simulink model "main"  (R2015a)
settings: Solver=ode1  StartTime=0.0  StopTime=Inf  FixedStep=0.001  RelTol=1e-3
PostLoadFcn:
  | , if any(exist('dsrtsu_mdlpostloadfcn', 'file') == [2, 3, 6]), try dsrtsu_mdlpostloadfcn('Execute', bdroot); catch fprintf('Error in PostLoadFcn (dsrtsu_mdlpostloadfcn) for model "%s":\n %s\n', bdroot, lasterr); end, end,
libraries: rtilibm x3, simulink_extras x3
settings Model: DSRTSU_INTERNAL_RTI_VER=460  DSRTSU_INTERNAL_RTI_TYPE=rti1005  DSRTSU_INTERNAL_RTIFPGA=50  Creator=k19p1400a  LastModifiedBy=k19p1400a
settings OptimizationCC: BlockReduction=off  OptimizeBlockIOStorage=off  BufferReuse=off  GlobalBufferReuse=off  ExpressionFolding=off  LocalBlockOutputs=off
settings HardwareCC: ProdIntDivRoundTo=Zero  ProdEndianess=BigEndian  ProdHWDeviceType=Generic->Custom  TargetIntDivRoundTo=Zero  TargetEndianess=BigEndian  TargetHWDeviceType=Generic->Custom
settings RTWCC: SystemTargetFile=rti1005.tlc  MakeCommand=make_rti  TemplateMakefile=rti1005.tmf  Description=dSPACE DS1005 Hardware Platform
settings STFCustomTargetCC: GenerateSampleERTMain=off  ParMdlRefBuildCompliant=on  GeneratePreprocessorConditionals=Disable all  ERTCustomFileBanners=off  SupportNonInlinedSFcns=on  SupportVariableSizeSignals=off  MATLABClassNameForMDSCustomization=Simulink.SoftwareTarget.GRTCustomization  GRTInterface=on  SystemTargetFile=rti1005.tlc
settings GRTTargetCC: CompOptLevelCompliant=off  ConcurrentExecutionCompliant=off  CombineOutputUpdateFcns=off  MatFileLogging=off  CPPClassGenCompliant=off  GRTInterface=on  ExtModeMexFile=noextcomm

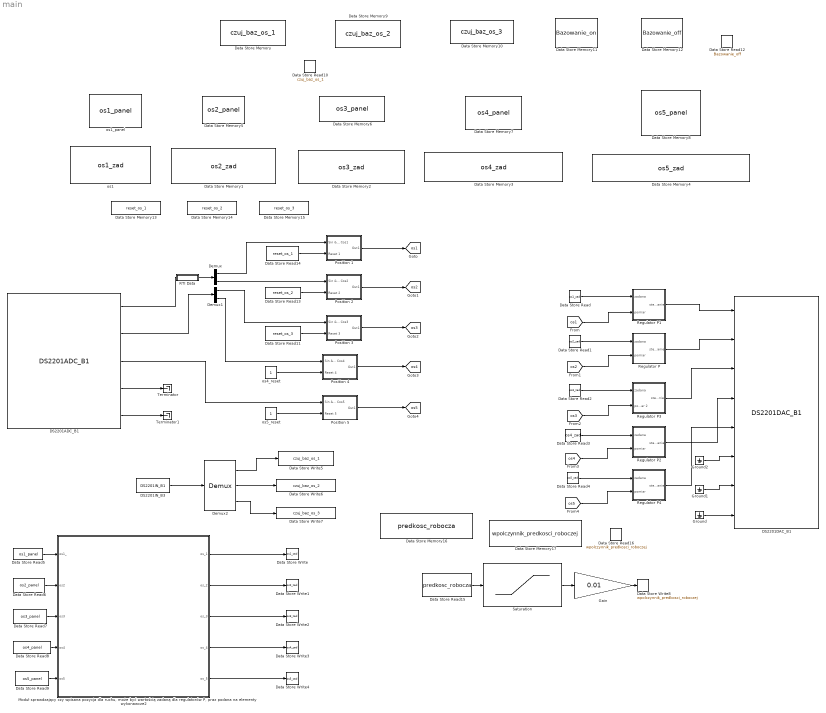
== system main ==
  DS2201ADC_B1 : rtilibm/DS2201/DS2201ADC_B1  BoardNo=1  channelNo1=[1 2 3 4]  channelNo2=[5 6 7 8]  channelNo3=[9 10]  channelNo4=-1  channelNo5=-1  DialogFcn=gui2201adc  UnitName={'DS2201ADC_B'}  UnitValues={ 1 }  DSProperties=struct('RTI',struct('Version',uint32(1),'BlockType',struct('isSLSource',uint8(1),'isSLSink',uint8(0),'isHWSource',uint8(1),'isHWSink',uint8(0),'isSetup',uint8(0),'isInline',uint8(1),'isNonInline',uint8(0),'isInterrupt',uint8(0),'isChannelwise',uint8(0)),'IOBoardType','DS2201','UnitType','ADC','Identifier','ADCMUX','DialogType','ML','BlockSet','NONE','SlaveProcessor','NONE'))
  DS2201DAC_B1 : rtilibm/DS2201/DS2201DAC_B1  BoardNo=1  IOErrorMode=[0 0]  InitValue=[0 0 0 0 0 0 0 0]  TermMode=[0 0 0 0 0 0 0 0]  TermValue=[0 0 0 0 0 0 0 0]  DialogFcn=gui2201dac  UnitName={'DS2201DAC_B'}  UnitValues={ 1 }  DSProperties=struct('RTI',struct('Version',uint32(1),'BlockType',struct('isSLSource',uint8(0),'isSLSink',uint8(1),'isHWSource',uint8(0),'isHWSink',uint8(1),'isSetup',uint8(0),'isInline',uint8(1),'isNonInline',uint8(0),'isInterrupt',uint8(0),'isChannelwise',uint8(0)),'IOBoardType','DS2201','UnitType','DAC','Identifier','DAC','DialogType','ML','BlockSet','NONE','SlaveProcessor','NONE'))
  DS2201IN_B3 : rtilibm/DS2201/DS2201IN_B1  BoardNo=3  ChannelNos=[1 2 3]  DialogFcn=gui2201in  UnitName={ 'DS2201IN_B' }  UnitValues={ 3 }  DSProperties=struct('RTI',struct('Version',uint32(1),'BlockType',struct('isSLSource',uint8(1),'isSLSink',uint8(0),'isHWSource',uint8(1),'isHWSink',uint8(0),'isSetup',uint8(0),'isInline',uint8(1),'isNonInline',uint8(0),'isInterrupt',uint8(0),'isChannelwise',uint8(0)),'IOBoardType','DS2201','UnitType','BIT','Identifier','BITIN','DialogType','ML','BlockSet','NONE','SlaveProcessor','NONE'))
  Data Store Memory : DataStoreMemory  DataStoreName=czuj_baz_os_1  ReadBeforeWriteMsg=warning  WriteAfterWriteMsg=warning  WriteAfterReadMsg=warning
  Data Store Memory1 : DataStoreMemory  DataStoreName=os2_zad  ReadBeforeWriteMsg=warning  WriteAfterWriteMsg=warning  WriteAfterReadMsg=warning
  Data Store Memory10 : DataStoreMemory  DataStoreName=czuj_baz_os_3  ReadBeforeWriteMsg=warning  WriteAfterWriteMsg=warning  WriteAfterReadMsg=warning
  Data Store Memory11 : DataStoreMemory  DataStoreName=Bazowanie_on  ReadBeforeWriteMsg=warning  WriteAfterWriteMsg=warning  WriteAfterReadMsg=warning  OutDataTypeStr=double
  Data Store Memory12 : DataStoreMemory  DataStoreName=Bazowanie_off  ReadBeforeWriteMsg=warning  WriteAfterWriteMsg=warning  WriteAfterReadMsg=warning  OutDataTypeStr=double
  Data Store Memory13 : DataStoreMemory  DataStoreName=reset_os_1  ReadBeforeWriteMsg=warning  WriteAfterWriteMsg=warning  WriteAfterReadMsg=warning
  Data Store Memory14 : DataStoreMemory  DataStoreName=reset_os_2  ReadBeforeWriteMsg=warning  WriteAfterWriteMsg=warning  WriteAfterReadMsg=warning
  Data Store Memory15 : DataStoreMemory  DataStoreName=reset_os_3  ReadBeforeWriteMsg=warning  WriteAfterWriteMsg=warning  WriteAfterReadMsg=warning
  Data Store Memory16 : DataStoreMemory  DataStoreName=predkosc_robocza  ReadBeforeWriteMsg=warning  WriteAfterWriteMsg=warning  WriteAfterReadMsg=warning
  Data Store Memory17 : DataStoreMemory  DataStoreName=wpolczynnik_predkosci_roboczej  ReadBeforeWriteMsg=warning  WriteAfterWriteMsg=warning  WriteAfterReadMsg=warning
  Data Store Memory2 : DataStoreMemory  DataStoreName=os3_zad  ReadBeforeWriteMsg=warning  WriteAfterWriteMsg=warning  WriteAfterReadMsg=warning
  Data Store Memory3 : DataStoreMemory  DataStoreName=os4_zad  ReadBeforeWriteMsg=warning  WriteAfterWriteMsg=warning  WriteAfterReadMsg=warning
  Data Store Memory4 : DataStoreMemory  DataStoreName=os5_zad  ReadBeforeWriteMsg=warning  WriteAfterWriteMsg=warning  WriteAfterReadMsg=warning
  Data Store Memory5 : DataStoreMemory  DataStoreName=os2_panel  ReadBeforeWriteMsg=warning  WriteAfterWriteMsg=warning  WriteAfterReadMsg=warning
  Data Store Memory6 : DataStoreMemory  DataStoreName=os3_panel  ReadBeforeWriteMsg=warning  WriteAfterWriteMsg=warning  WriteAfterReadMsg=warning
  Data Store Memory7 : DataStoreMemory  DataStoreName=os4_panel  ReadBeforeWriteMsg=warning  WriteAfterWriteMsg=warning  WriteAfterReadMsg=warning
  Data Store Memory8 : DataStoreMemory  DataStoreName=os5_panel  ReadBeforeWriteMsg=warning  WriteAfterWriteMsg=warning  WriteAfterReadMsg=warning
  Data Store Memory9 : DataStoreMemory  DataStoreName=czuj_baz_os_2  ReadBeforeWriteMsg=warning  WriteAfterWriteMsg=warning  WriteAfterReadMsg=warning
  Data Store Read : DataStoreRead  DataStoreName=os1_zad
  Data Store Read1 : DataStoreRead  DataStoreName=os2_zad
  Data Store Read10 : DataStoreRead  DataStoreName=czuj_baz_os_1
  Data Store Read11 : DataStoreRead  DataStoreName=reset_os_3
  Data Store Read12 : DataStoreRead  DataStoreName=Bazowanie_off
  Data Store Read13 : DataStoreRead  DataStoreName=reset_os_2
  Data Store Read14 : DataStoreRead  DataStoreName=reset_os_1
  Data Store Read15 : DataStoreRead  DataStoreName=predkosc_robocza
  Data Store Read16 : DataStoreRead  DataStoreName=wpolczynnik_predkosci_roboczej
  Data Store Read2 : DataStoreRead  DataStoreName=os3_zad
  Data Store Read3 : DataStoreRead  DataStoreName=os4_zad
  Data Store Read4 : DataStoreRead  DataStoreName=os5_zad
  Data Store Read5 : DataStoreRead  DataStoreName=os1_panel
  Data Store Read6 : DataStoreRead  DataStoreName=os2_panel
  Data Store Read7 : DataStoreRead  DataStoreName=os3_panel
  Data Store Read8 : DataStoreRead  DataStoreName=os4_panel
  Data Store Read9 : DataStoreRead  DataStoreName=os5_panel
  Data Store Write : DataStoreWrite  DataStoreName=os1_zad
  Data Store Write1 : DataStoreWrite  DataStoreName=os2_zad
  Data Store Write2 : DataStoreWrite  DataStoreName=os3_zad
  Data Store Write3 : DataStoreWrite  DataStoreName=os4_zad
  Data Store Write4 : DataStoreWrite  DataStoreName=os5_zad
  Data Store Write5 : DataStoreWrite  DataStoreName=czuj_baz_os_1
  Data Store Write6 : DataStoreWrite  DataStoreName=czuj_baz_os_2
  Data Store Write7 : DataStoreWrite  DataStoreName=czuj_baz_os_3
  Data Store Write8 : DataStoreWrite  DataStoreName=wpolczynnik_predkosci_roboczej
  Demux : Demux  Outputs=2
  Demux1 : Demux  Outputs=2
  Demux2 : Demux  Outputs=3
  Gain : Gain  Gain=0.01
  Ground : Ground
  Ground1 : Ground
  Ground2 : Ground
  "Moduł sprawdzający czy wpisana pozycja dla ruchu, może być wartością zadaną dla regulatorów P, praz podana na elementy wykonawcze2" : Subsystem
  Position 1 : Subsystem
  Position 2 : Subsystem
  Position 3 : Subsystem
  Position 4 : Subsystem
  Position 5 : Subsystem
  RTI Data : Subsystem  Tag=struct('RTIDataServer',struct('RTIDataServerVs','2','RTIModelDescription','struct(''main'',''main'',''sub'',''main'',''isMp'',0)'))  LoadFcn="if exist('rtidc'), try,  rtidc('DataHostBlockClbLoad', gcbh); catch, disp(['Warning: ''LoadFcn'' for RTI Data block failed: ' lasterr]); end, end,"  mask(RTI_DATA_HOST){}
      mask help:
      | RTI Data Block.
      | This block is used by RTI to store internal model-dependent data.
      | Please keep this block on the root level of the model. Deleting this block will result in data loss.
      |
      | NEVER DELETE OR COPY THIS BLOCK!
      settings: CopyFcn="if exist('rtidc'), try,  rtidc('DataHostBlockClbCopy', gcbh); catch, disp(['Warning: ''CopyFcn'' for RTI Data block failed: ' lasterr]); end, end,"  DeleteFcn="if exist('rtidc'), try,  rtidc('DataHostBlockClbDelete', gcbh); catch, disp(['Warning: ''DeleteFcn'' for RTI Data block failed: ' lasterr]); end, end,"  ModelCloseFcn="if exist('rtidc'), try,  rtidc('DataHostBlockClbModelClose', gcbh); catch, disp(['Warning: ''ModelCloseFcn'' for RTI Data block failed: ' lasterr]); end, end,"  PreSaveFcn="if exist('rtidc'), try,  rtidc('DataHostBlockClbPreSave', gcbh); catch, disp(['Warning: ''PreSaveFcn'' for RTI Data block failed: ' lasterr]); end, end,"  PostSaveFcn="if exist('rtidc'), try,  rtidc('DataHostBlockClbPostSave', gcbh); catch, disp(['Warning: ''PostSaveFcn'' for RTI Data block failed: ' lasterr]); end, end,"  NameChangeFcn="if exist('rtidc'), try,  rtidc('DataHostBlockClbNameChange', gcbh); catch, disp(['Warning: ''NameChangeFcn'' for RTI Data block failed: ' lasterr]); end, end,"
      mask Help:
      | RTI Data Block.
      | This block is used by RTI to store internal model-dependent data.
      | Please keep this block on the root level of the model. Deleting this block will result in data loss.
      | 
      | NEVER DELETE OR COPY THIS BLOCK!
      mask Display:
      | text(0.5, 0.5, 'RTI Data', 'HorizontalAlignment', 'center');
      | plot([1 0]);
  Regulator P : Subsystem
  Regulator P1 : Subsystem
  Regulator P2 : Subsystem
  Regulator P3 : Subsystem
  Regulator P4 : Subsystem
  Saturation : Saturate  UpperLimit=100  LowerLimit=5
  Terminator : Terminator
  Terminator1 : Terminator
  os1 : DataStoreMemory  DataStoreName=os1_zad  ReadBeforeWriteMsg=warning  WriteAfterWriteMsg=warning  WriteAfterReadMsg=warning
  "os1_panel " : DataStoreMemory  DataStoreName=os1_panel  ReadBeforeWriteMsg=warning  WriteAfterWriteMsg=warning  WriteAfterReadMsg=warning
  os4_reset : Constant  OutDataTypeStr=double
  "os5_reset " : Constant  OutDataTypeStr=double
  tag scope: os1=global, os2=global, os3=global, os4=global, os5=global
  wires:
  Position 1/1(Out1) -> [os1]
  Position 2/1(Out1) -> [os2]
  Position 3/1(Out1) -> [os3]
  Position 5/1(Out1) -> [os5]
  Position 4/1(Out1) -> [os4]
  DS2201ADC_B1/5 -> Terminator1/1
  DS2201ADC_B1/4 -> Terminator/1
  DS2201ADC_B1/2 -> Demux1/1
  DS2201ADC_B1/1 -> Demux/1
  Demux/1 -> Position 1/1(Sin && Cos1)
  Demux/2 -> Position 2/1(Sin && Cos2)
  Demux1/1 -> Position 3/1(Sin && Cos3)
  Demux1/2 -> Position 4/1(Sin && Cos4)
  DS2201ADC_B1/3 -> Position 5/1(Sin && Cos5)
  [os1] -> Regulator P1/2("pomiar ")
  [os2] -> Regulator P/2("pomiar ")
  [os4] -> Regulator P2/2("pomiar ")
  [os5] -> Regulator P4/2("pomiar ")
  Data Store Read/1 -> Regulator P1/1(zadana)
  Regulator P1/1(sterowanie) -> DS2201DAC_B1/1
  Regulator P/1(sterowanie) -> DS2201DAC_B1/2
  Regulator P2/1(sterowanie) -> DS2201DAC_B1/4
  Regulator P4/1(sterowanie) -> DS2201DAC_B1/5
  Data Store Read4/1 -> Regulator P4/1(zadana)
  Data Store Read3/1 -> Regulator P2/1(zadana)
  Data Store Read1/1 -> Regulator P/1(zadana)
  "os5_reset "/1 -> Position 5/2(Reset 5)
  os4_reset/1 -> Position 4/2(Reset 4)
  Data Store Read11/1 -> Position 3/2(Reset 3)
  Data Store Read13/1 -> Position 2/2(Reset 2)
  DS2201IN_B3/1 -> Demux2/1
  Ground/1 -> DS2201DAC_B1/8
  Ground1/1 -> DS2201DAC_B1/7
  Ground2/1 -> DS2201DAC_B1/6
  "Moduł sprawdzający czy wpisana pozycja dla ruchu, może być wartością zadaną dla regulatorów P, praz podana na elementy wykonawcze2"/3(os_3) -> Data Store Write2/1
  "Moduł sprawdzający czy wpisana pozycja dla ruchu, może być wartością zadaną dla regulatorów P, praz podana na elementy wykonawcze2"/2(os_2) -> Data Store Write1/1
  "Moduł sprawdzający czy wpisana pozycja dla ruchu, może być wartością zadaną dla regulatorów P, praz podana na elementy wykonawcze2"/4(os_4) -> Data Store Write3/1
  "Moduł sprawdzający czy wpisana pozycja dla ruchu, może być wartością zadaną dla regulatorów P, praz podana na elementy wykonawcze2"/1(os_1) -> Data Store Write/1
  "Moduł sprawdzający czy wpisana pozycja dla ruchu, może być wartością zadaną dla regulatorów P, praz podana na elementy wykonawcze2"/5(os_5) -> Data Store Write4/1
  Data Store Read6/1 -> "Moduł sprawdzający czy wpisana pozycja dla ruchu, może być wartością zadaną dla regulatorów P, praz podana na elementy wykonawcze2"/2(os2)
  Data Store Read5/1 -> "Moduł sprawdzający czy wpisana pozycja dla ruchu, może być wartością zadaną dla regulatorów P, praz podana na elementy wykonawcze2"/1(os1_)
  Data Store Read7/1 -> "Moduł sprawdzający czy wpisana pozycja dla ruchu, może być wartością zadaną dla regulatorów P, praz podana na elementy wykonawcze2"/3(os3)
  Data Store Read8/1 -> "Moduł sprawdzający czy wpisana pozycja dla ruchu, może być wartością zadaną dla regulatorów P, praz podana na elementy wykonawcze2"/4(os4)
  Data Store Read9/1 -> "Moduł sprawdzający czy wpisana pozycja dla ruchu, może być wartością zadaną dla regulatorów P, praz podana na elementy wykonawcze2"/5(os5)
  Demux2/1 -> Data Store Write5/1
  Demux2/2 -> Data Store Write6/1
  Demux2/3 -> Data Store Write7/1
  Data Store Read14/1 -> Position 1/2(Reset 1)
  Data Store Read2/1 -> Regulator P3/1(zadana)
  [os3] -> Regulator P3/2(pomiar 2)
  Regulator P3/1(sterowanie) -> DS2201DAC_B1/3
  Data Store Read15/1 -> Saturation/1
  Saturation/1 -> Gain/1
  Gain/1 -> Data Store Write8/1

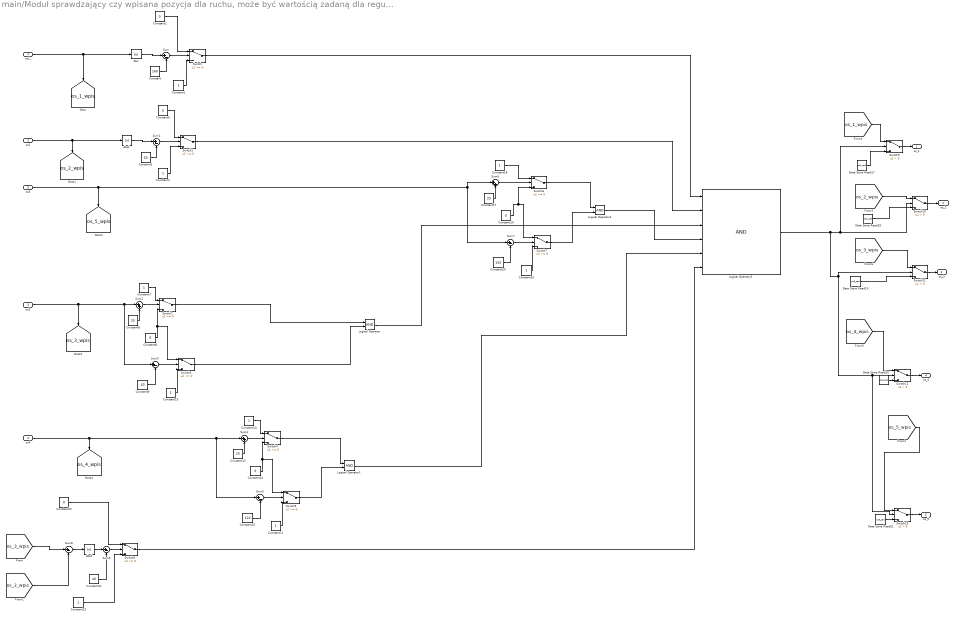
== system main/Moduł sprawdzający czy wpisana pozycja dla ruchu, może być wartością zadaną dla regulatorów P, praz podana na elementy wykonawcze2 ==
  os1_ : Inport
  os2 : Inport  Port=2
  os3 : Inport  Port=3
  os4 : Inport  Port=4
  os5 : Inport  Port=5
  Abs : Abs
  Abs1 : Abs
  Abs2 : Abs
  Constant : Constant  Value=160
  Constant{1,4,7,10..11,13,16,18,23} (9 alike) : Constant
  Constant12 : Constant  Value=25
  Constant{2,5,8,14,19,22} (6 alike) : Constant  Value=0
  Constant15 : Constant  Value=120
  Constant17 : Constant  Value=25
  Constant20 : Constant  Value=150
  Constant21 : Constant  Value=40
  Constant3 : Constant  Value=40
  Constant6 : Constant  Value=25
  Constant9 : Constant  Value=40
  Data Store Read17 : DataStoreRead  DataStoreName=os1_zad
  Data Store Read18 : DataStoreRead  DataStoreName=os2_zad
  Data Store Read19 : DataStoreRead  DataStoreName=os3_zad
  Data Store Read20 : DataStoreRead  DataStoreName=os4_zad
  Data Store Read21 : DataStoreRead  DataStoreName=os5_zad
  Logical Operator : Logic  AllPortsSameDT=off
  Logical Operator1 : Logic  AllPortsSameDT=off
  Logical Operator2 : Logic  AllPortsSameDT=off
  Logical Operator3 : Logic  Inputs=6  AllPortsSameDT=off
  Sum{,1,3,5,7..9} (7 alike) : Sum  Inputs=|+-
  Sum2 : Sum  Inputs=|++
  Sum4 : Sum  Inputs=|++
  Sum6 : Sum  Inputs=|++
  Switch{,1..8} (9 alike) : Switch
  Switch{9..13} (5 alike) : Switch  Criteria=u2 > Threshold
  os_1 : Outport
  os_2 : Outport  Port=2
  os_3 : Outport  Port=3
  os_4 : Outport  Port=4
  os_5 : Outport  Port=5
  tag scope: os_1_wpis=global, os_2_wpis=global, os_3_wpis=global, os_4_wpis=global, os_5_wpis=global
  wires:
  Constant18/1 -> Switch6/1
  Data Store Read19/1 -> Switch11/3
  [os_3_wpis] -> Switch11/1
  os3/1 -> Sum3/1, Sum2/1, [os_3_wpis]
  Sum2/1 -> Switch2/2
  Switch8/1 -> Logical Operator3/6
  Abs/1 -> Sum/1
  Abs2/1 -> Sum9/1
  os2/1 -> Abs1/1, [os_2_wpis]
  Switch7/1 -> Logical Operator2/2
  Logical Operator/1 -> Logical Operator3/3
  Constant21/1 -> Sum9/2
  Constant20/1 -> Sum7/2
  Constant10/1 -> Switch3/3
  Switch5/1 -> Logical Operator1/2
  Constant3/1 -> Sum1/2
  [os_2_wpis] -> Switch10/1
  Sum6/1 -> Switch6/2
  Constant19/1 -> Switch7/1, Switch6/3
  Sum8/1 -> Abs2/1
  Constant16/1 -> Switch7/3
  Constant1/1 -> Switch/3
  Logical Operator2/1 -> Logical Operator3/4
  Sum/1 -> Switch/2
  os5/1 -> [os_5_wpis], Sum6/1, Sum7/1
  Constant7/1 -> Switch2/1
  Constant14/1 -> Switch5/1, Switch4/3
  Logical Operator1/1 -> Logical Operator3/5
  [os_5_wpis] -> Switch13/1
  Switch6/1 -> Logical Operator2/1
  [os_4_wpis] -> Switch12/1
  Sum7/1 -> Switch7/2
  Data Store Read20/1 -> Switch12/3
  Switch1/1 -> Logical Operator3/2
  Constant8/1 -> Switch3/1, Switch2/3
  Abs1/1 -> Sum1/1
  [os_1_wpis] -> Switch9/1
  Constant9/1 -> Sum3/2
  Constant6/1 -> Sum2/2
  Constant/1 -> Sum/2
  Switch/1 -> Logical Operator3/1
  Data Store Read17/1 -> Switch9/3
  Data Store Read21/1 -> Switch13/3
  Data Store Read18/1 -> Switch10/3
  Switch4/1 -> Logical Operator1/1
  Sum5/1 -> Switch5/2
  Constant5/1 -> Switch1/1
  Logical Operator3/1 -> Switch13/2, Switch12/2, Switch11/2, Switch10/2, Switch9/2
  Constant22/1 -> Switch8/1
  Constant4/1 -> Switch1/3
  Constant2/1 -> Switch/1
  Constant13/1 -> Switch4/1
  Sum3/1 -> Switch3/2
  Switch3/1 -> Logical Operator/2
  Sum4/1 -> Switch4/2
  os4/1 -> [os_4_wpis], Sum4/1, Sum5/1
  Switch2/1 -> Logical Operator/1
  Constant11/1 -> Switch5/3
  Constant17/1 -> Sum6/2
  Constant12/1 -> Sum4/2
  Constant15/1 -> Sum5/2
  Sum9/1 -> Switch8/2
  Constant23/1 -> Switch8/3
  Sum1/1 -> Switch1/2
  os1_/1 -> [os_1_wpis], Abs/1
  Switch9/1 -> os_1/1
  Switch10/1 -> os_2/1
  Switch11/1 -> os_3/1
  Switch12/1 -> os_4/1
  Switch13/1 -> os_5/1
  [os_3_wpis] -> Sum8/1
  [os_2_wpis] -> Sum8/2

== system main/Position 1 ==
  Sin && Cos1 : Inport
  Reset 1 : Inport  Port=2
  Filters 1 : Subsystem
  Position Calculation 1 : Subsystem
  Out1 : Outport
  wires:
  Position Calculation 1/1(Position) -> Out1/1
  Reset 1/1 -> Position Calculation 1/3(Reset (Impulse))
  Sin && Cos1/1 -> Filters 1/1(Sin && Cos)
  Filters 1/2(Cos) -> Position Calculation 1/2(Cos)
  Filters 1/1(Sin) -> Position Calculation 1/1(Sin)

== system main/Position 2 ==
  Sin && Cos2 : Inport
  Reset 2 : Inport  Port=2
  Filters 2 : Subsystem
  Position Calculation 2 : Subsystem
  Out1 : Outport
  wires:
  Position Calculation 2/1(Position) -> Out1/1
  Reset 2/1 -> Position Calculation 2/3(Reset (Impulse))
  Sin && Cos2/1 -> Filters 2/1(Sin && Cos)
  Filters 2/2(Cos) -> Position Calculation 2/2(Cos)
  Filters 2/1(Sin) -> Position Calculation 2/1(Sin)

== system main/Position 3 ==
  Sin && Cos3 : Inport
  Reset 3 : Inport  Port=2
  Filters 3 : Subsystem
  Position Calculation 3 : Subsystem
  Out1 : Outport
  wires:
  Position Calculation 3/1(Position) -> Out1/1
  Reset 3/1 -> Position Calculation 3/3(Reset (Impulse))
  Sin && Cos3/1 -> Filters 3/1(Sin && Cos)
  Filters 3/2(Cos) -> Position Calculation 3/2(Cos)
  Filters 3/1(Sin) -> Position Calculation 3/1(Sin)

== system main/Position 4 ==
  Sin && Cos4 : Inport
  Reset 4 : Inport  Port=2
  Filters 4 : Subsystem
  Position Calculation 4 : Subsystem
  Out1 : Outport
  wires:
  Filters 4/1(Sin) -> Position Calculation 4/1(Sin)
  Filters 4/2(Cos) -> Position Calculation 4/2(Cos)
  Sin && Cos4/1 -> Filters 4/1(Sin && Cos)
  Reset 4/1 -> Position Calculation 4/3(Reset (Impulse))
  Position Calculation 4/1(Position) -> Out1/1

== system main/Position 5 ==
  Sin && Cos5 : Inport
  Reset 5 : Inport  Port=2
  Filters 5 : Subsystem
  Position Calculation 5 : Subsystem
  Out1 : Outport
  wires:
  Filters 5/1(Sin) -> Position Calculation 5/1(Sin)
  Filters 5/2(Cos) -> Position Calculation 5/2(Cos)
  Sin && Cos5/1 -> Filters 5/1(Sin && Cos)
  Reset 5/1 -> Position Calculation 5/3(Reset (Impulse))
  Position Calculation 5/1(Position) -> Out1/1

== system main/RTI Data ==
  RTI Data Store : Subsystem  Tag="struct('private',struct('version',struct('dsVer',uint32(2),'dsVerCreation',uint32(2),'RTI',struct('ver','7.4','type','RTI1005')),'access',struct('type','Model','isPerm',1,'created',['11-Mar-2019 14:33:50'],'modified',['18-Mar-2019 15:29:44'],'location','')),'public',struct('main',struct('data',[]),'sub',struct('name',{{'main'}},'data',{{struct('TH',struct('thTaskInfo',struct('taskType',{'TIMER','HWINT','TMRINT','SWINT','GLINT'},'tasksNumOf',{1,0,0,0,0},'srcIds',{{'TIMERA'},{},{},{},{}},'taskNames',{{['Timer Task 1']},{},{},{},{}})),'th_tc',struct('dataType','TASK','taskGroupId','','taskGroupList',{{}},'taskSchedulingPolicy','FCFS','taskType','TIMER','blkh',-1,'srcId','TIMERA','srcSgnName',['Timer A interrupt'],'srcCpuName','','taskName',['Timer Task 1  [0.001] s'],'taskNameDisplayExt','','smplTime',0.001,'smplTimeOffs',0,'hasFixedPriority',0,'priority',1,'hasFixedOvc',0,'ovcType',1,'ovcMax',1),'tc_th',struct('dataType','TASK','taskGroupId','','taskGroupList',{{}},'taskSchedulingPolicy','FCFS','taskType','TIMER','blkh',-1,'srcId','TIMERA','srcSgnName',['Timer A interrupt'],'srcCpuName','','taskName',['Timer Task 1  [0.001] s'],'taskNameDisplayExt','','smplTime',0.001,'smplTimeOffs',0,'hasFixedPriority',0,'priority',1,'hasFixedOvc',0,'ovcType',1,'ovcMax',1))}})))"  mask(RTI_DATA_STORE){}
      mask help:
      | RTI Data Store Block. This block is used by RTI to store internal model dependent data. Deleting this block will result in data loss.
      |
      | NEVER DELETE, COPY, OR MODIFY THIS BLOCK!
      mask Help:
      | RTI Data Store Block. This block is used by RTI to store internal model dependent data. Deleting this block will result in data loss.
      | 
      | NEVER DELETE, COPY, OR MODIFY THIS BLOCK!
      mask Display: text(0.5, 0.5, ' ', 'HorizontalAlignment', 'center');

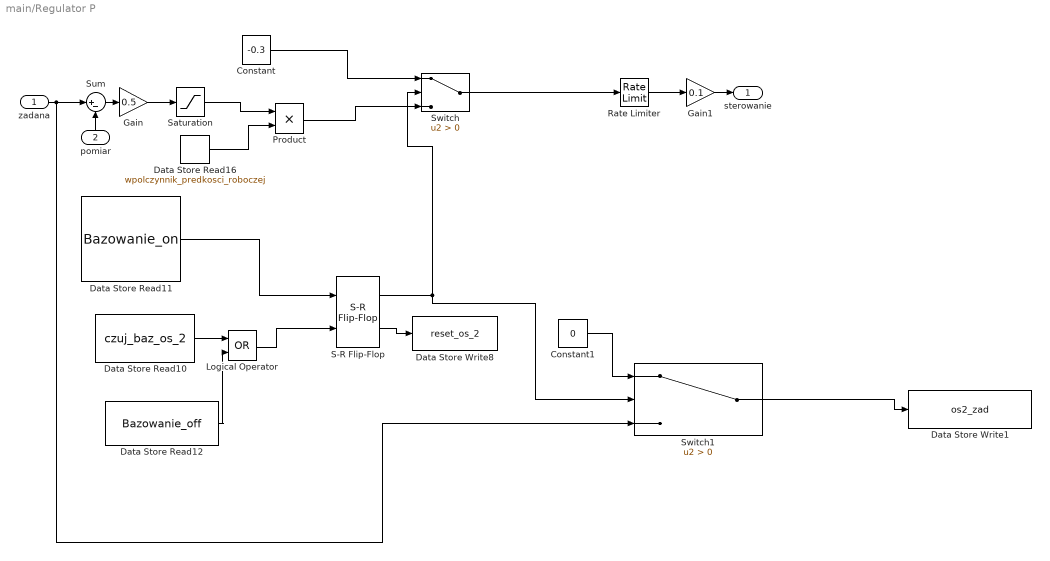
== system main/Regulator P ==
  zadana : Inport
  "pomiar " : Inport  Port=2
  Constant : Constant  Value=-0.3
  Constant1 : Constant  Value=0
  Data Store Read10 : DataStoreRead  DataStoreName=czuj_baz_os_2
  Data Store Read11 : DataStoreRead  DataStoreName=Bazowanie_on
  Data Store Read12 : DataStoreRead  DataStoreName=Bazowanie_off
  Data Store Read16 : DataStoreRead  DataStoreName=wpolczynnik_predkosci_roboczej
  Data Store Write1 : DataStoreWrite  DataStoreName=os2_zad
  Data Store Write8 : DataStoreWrite  DataStoreName=reset_os_2
  Gain : Gain  Gain=0.5
  Gain1 : Gain  Gain=0.1
  Logical Operator : Logic  Operator=OR  AllPortsSameDT=off
  Product : Product
  Rate Limiter : RateLimiter  RisingSlewLimit=50  FallingSlewLimit=-50  SampleTimeMode=inherited
  S-R Flip-Flop : simulink_extras/Flip Flops/S-R Flip-Flop  initial_condition=0
  Saturation : Saturate  UpperLimit=3  LowerLimit=-3
  Sum : Sum  Inputs=|+-
  Switch : Switch  Criteria=u2 > Threshold
  Switch1 : Switch  Criteria=u2 > Threshold
  sterowanie : Outport
  wires:
  Gain/1 -> Saturation/1
  Gain1/1 -> sterowanie/1
  "pomiar "/1 -> Sum/2
  Rate Limiter/1 -> Gain1/1
  Sum/1 -> Gain/1
  zadana/1 -> Switch1/3, Sum/1
  Data Store Read10/1 -> Logical Operator/1
  Data Store Read12/1 -> Logical Operator/2
  S-R Flip-Flop/2 -> Data Store Write8/1
  S-R Flip-Flop/1 -> Switch/2, Switch1/2
  Constant1/1 -> Switch1/1
  Logical Operator/1 -> S-R Flip-Flop/2
  Data Store Read11/1 -> S-R Flip-Flop/1
  Constant/1 -> Switch/1
  Switch/1 -> Rate Limiter/1
  Switch1/1 -> Data Store Write1/1
  Saturation/1 -> Product/1
  Data Store Read16/1 -> Product/2
  Product/1 -> Switch/3

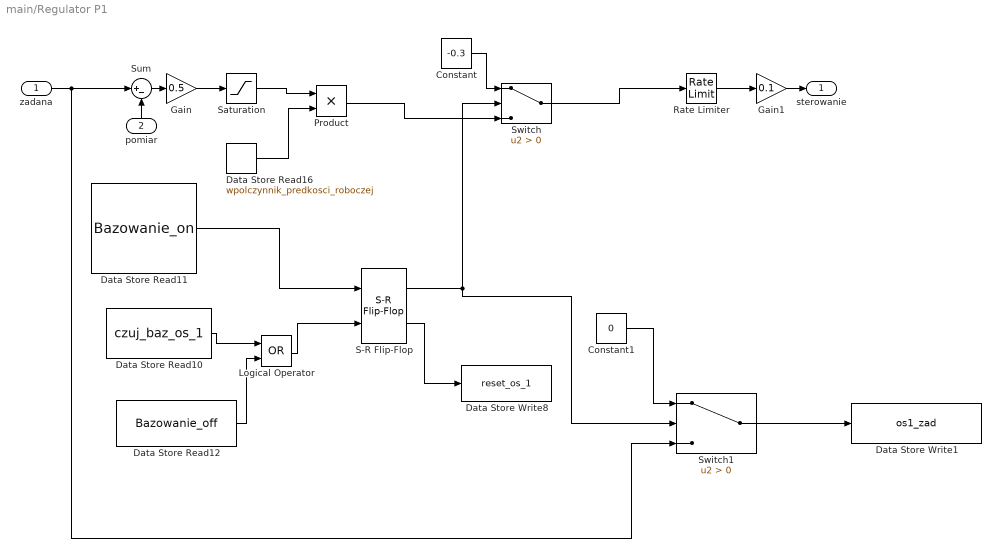
== system main/Regulator P1 ==
  zadana : Inport
  "pomiar " : Inport  Port=2
  Constant : Constant  Value=-0.3
  Constant1 : Constant  Value=0
  Data Store Read10 : DataStoreRead  DataStoreName=czuj_baz_os_1
  Data Store Read11 : DataStoreRead  DataStoreName=Bazowanie_on
  Data Store Read12 : DataStoreRead  DataStoreName=Bazowanie_off
  Data Store Read16 : DataStoreRead  DataStoreName=wpolczynnik_predkosci_roboczej
  Data Store Write1 : DataStoreWrite  DataStoreName=os1_zad
  Data Store Write8 : DataStoreWrite  DataStoreName=reset_os_1
  Gain : Gain  Gain=0.5
  Gain1 : Gain  Gain=0.1
  Logical Operator : Logic  Operator=OR  AllPortsSameDT=off
  Product : Product
  Rate Limiter : RateLimiter  RisingSlewLimit=50  FallingSlewLimit=-50  SampleTimeMode=inherited
  S-R Flip-Flop : simulink_extras/Flip Flops/S-R Flip-Flop  initial_condition=0
  Saturation : Saturate  UpperLimit=3  LowerLimit=-3
  Sum : Sum  Inputs=|+-
  Switch : Switch  Criteria=u2 > Threshold
  Switch1 : Switch  Criteria=u2 > Threshold
  sterowanie : Outport
  wires:
  Gain/1 -> Saturation/1
  Gain1/1 -> sterowanie/1
  "pomiar "/1 -> Sum/2
  Rate Limiter/1 -> Gain1/1
  zadana/1 -> Switch1/3, Sum/1
  Sum/1 -> Gain/1
  Switch/1 -> Rate Limiter/1
  Constant/1 -> Switch/1
  Data Store Read10/1 -> Logical Operator/1
  Data Store Read12/1 -> Logical Operator/2
  S-R Flip-Flop/2 -> Data Store Write8/1
  S-R Flip-Flop/1 -> Switch/2, Switch1/2
  Constant1/1 -> Switch1/1
  Switch1/1 -> Data Store Write1/1
  Logical Operator/1 -> S-R Flip-Flop/2
  Data Store Read11/1 -> S-R Flip-Flop/1
  Saturation/1 -> Product/1
  Data Store Read16/1 -> Product/2
  Product/1 -> Switch/3

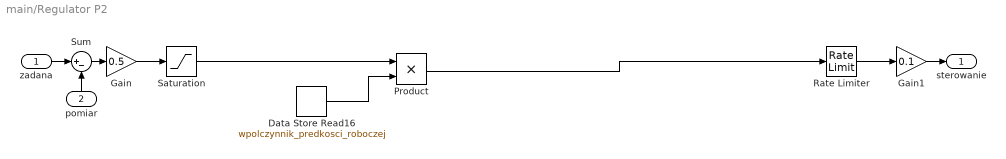
== system main/Regulator P2 ==
  zadana : Inport
  "pomiar " : Inport  Port=2
  Data Store Read16 : DataStoreRead  DataStoreName=wpolczynnik_predkosci_roboczej
  Gain : Gain  Gain=0.5
  Gain1 : Gain  Gain=0.1
  Product : Product
  Rate Limiter : RateLimiter  RisingSlewLimit=50  FallingSlewLimit=-50  SampleTimeMode=inherited
  Saturation : Saturate  UpperLimit=3  LowerLimit=-3
  Sum : Sum  Inputs=|+-
  sterowanie : Outport
  wires:
  Gain/1 -> Saturation/1
  Gain1/1 -> sterowanie/1
  "pomiar "/1 -> Sum/2
  Rate Limiter/1 -> Gain1/1
  zadana/1 -> Sum/1
  Sum/1 -> Gain/1
  Data Store Read16/1 -> Product/2
  Product/1 -> Rate Limiter/1
  Saturation/1 -> Product/1

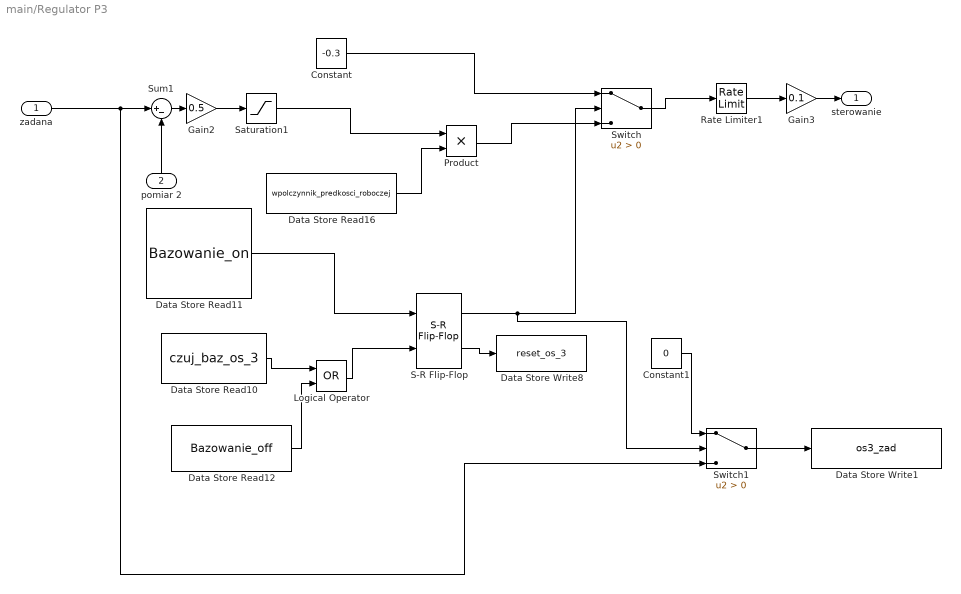
== system main/Regulator P3 ==
  zadana : Inport
  pomiar 2 : Inport  Port=2
  Constant : Constant  Value=-0.3
  Constant1 : Constant  Value=0
  Data Store Read10 : DataStoreRead  DataStoreName=czuj_baz_os_3
  Data Store Read11 : DataStoreRead  DataStoreName=Bazowanie_on
  Data Store Read12 : DataStoreRead  DataStoreName=Bazowanie_off
  Data Store Read16 : DataStoreRead  DataStoreName=wpolczynnik_predkosci_roboczej
  Data Store Write1 : DataStoreWrite  DataStoreName=os3_zad
  Data Store Write8 : DataStoreWrite  DataStoreName=reset_os_3
  Gain2 : Gain  Gain=0.5
  Gain3 : Gain  Gain=0.1
  Logical Operator : Logic  Operator=OR  AllPortsSameDT=off
  Product : Product
  Rate Limiter1 : RateLimiter  RisingSlewLimit=50  FallingSlewLimit=-50  SampleTimeMode=inherited
  S-R Flip-Flop : simulink_extras/Flip Flops/S-R Flip-Flop  initial_condition=0
  Saturation1 : Saturate  UpperLimit=3  LowerLimit=-3
  Sum1 : Sum  Inputs=|+-
  Switch : Switch  Criteria=u2 > Threshold
  Switch1 : Switch  Criteria=u2 > Threshold
  sterowanie : Outport
  wires:
  Gain2/1 -> Saturation1/1
  Gain3/1 -> sterowanie/1
  pomiar 2/1 -> Sum1/2
  Rate Limiter1/1 -> Gain3/1
  Sum1/1 -> Gain2/1
  zadana/1 -> Switch1/3, Sum1/1
  Data Store Read10/1 -> Logical Operator/1
  Data Store Read12/1 -> Logical Operator/2
  S-R Flip-Flop/2 -> Data Store Write8/1
  S-R Flip-Flop/1 -> Switch/2, Switch1/2
  Constant1/1 -> Switch1/1
  Logical Operator/1 -> S-R Flip-Flop/2
  Data Store Read11/1 -> S-R Flip-Flop/1
  Constant/1 -> Switch/1
  Switch/1 -> Rate Limiter1/1
  Switch1/1 -> Data Store Write1/1
  Data Store Read16/1 -> Product/2
  Product/1 -> Switch/3
  Saturation1/1 -> Product/1

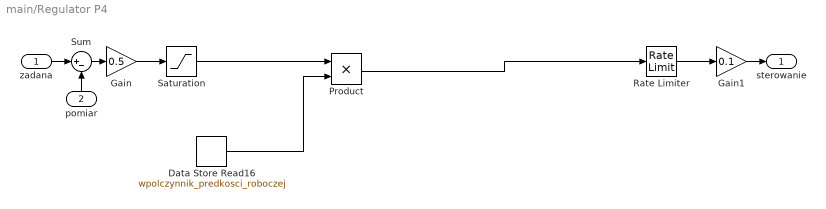
== system main/Regulator P4 ==
  zadana : Inport
  "pomiar " : Inport  Port=2
  Data Store Read16 : DataStoreRead  DataStoreName=wpolczynnik_predkosci_roboczej
  Gain : Gain  Gain=0.5
  Gain1 : Gain  Gain=0.1
  Product : Product
  Rate Limiter : RateLimiter  RisingSlewLimit=50  FallingSlewLimit=-50  SampleTimeMode=inherited
  Saturation : Saturate  UpperLimit=3  LowerLimit=-3
  Sum : Sum  Inputs=|+-
  sterowanie : Outport
  wires:
  Gain/1 -> Saturation/1
  Gain1/1 -> sterowanie/1
  "pomiar "/1 -> Sum/2
  Rate Limiter/1 -> Gain1/1
  zadana/1 -> Sum/1
  Sum/1 -> Gain/1
  Data Store Read16/1 -> Product/2
  Product/1 -> Rate Limiter/1
  Saturation/1 -> Product/1

== system main/Position 1/Filters 1 ==
  Sin && Cos : Inport
  Analog Butterworth LP Filter : Subsystem  mask(buttap){Parameter3=2*pi*16, Parameter4=1}
      mask prompts: Parameter3 "Cutoff frequency (rad/sec)"; Parameter4 "Order"
      mask help:
      | Analog Butterworth low pass filter.
      |
      | (Requires Signal Processing Toolbox)
      mask init:
      | [z,p,k]=buttap(@2); z=@1*z; p=@1*p; k=real(prod(-p)); [num,den]=zp2tf(z,p,k); w=logspace(log10(@1/10),log10(10*@1),20); h=freqs(num,den,w);
      mask Help: Butterworth low pass filter using MATLAB's butter command.
      mask Display: plot(20*log10(w),20*log10(abs(h)))
  Analog Butterworth LP Filter1 : Subsystem  mask(buttap){Parameter3=2*pi*16, Parameter4=1}
      mask prompts: Parameter3 "Cutoff frequency (rad/sec)"; Parameter4 "Order"
      mask help:
      | Analog Butterworth low pass filter.
      |
      | (Requires Signal Processing Toolbox)
      mask init:
      | [z,p,k]=buttap(@2); z=@1*z; p=@1*p; k=real(prod(-p)); [num,den]=zp2tf(z,p,k); w=logspace(log10(@1/10),log10(10*@1),20); h=freqs(num,den,w);
      mask Help: Butterworth low pass filter using MATLAB's butter command.
      mask Display: plot(20*log10(w),20*log10(abs(h)))
  Demux : Demux  Outputs=2
  Sin : Outport
  Cos : Outport  Port=2
  wires:
  Analog Butterworth LP Filter/1(Out1) -> Sin/1
  Analog Butterworth LP Filter1/1(Out1) -> Cos/1
  Sin && Cos/1 -> Demux/1
  Demux/1 -> Analog Butterworth LP Filter/1(In1)
  Demux/2 -> Analog Butterworth LP Filter1/1(In1)

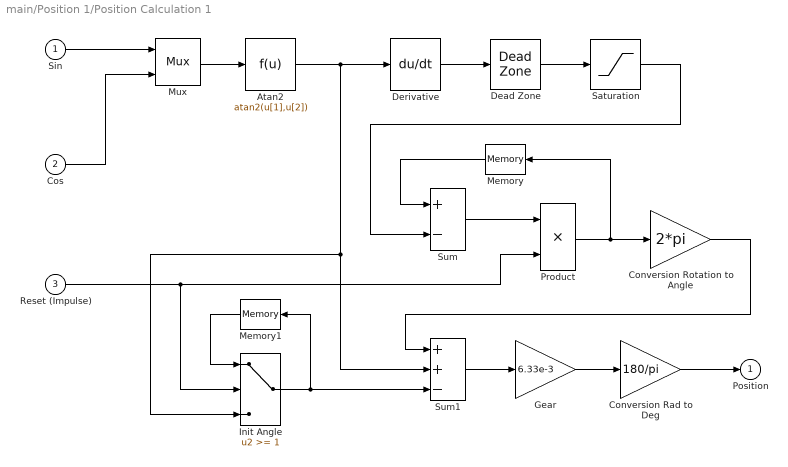
== system main/Position 1/Position Calculation 1 ==
  Sin : Inport
  Cos : Inport  Port=2
  Reset (Impulse) : Inport  Port=3
  Atan2 : Fcn  Expr=atan2(u[1],u[2])
  Conversion Rad to Deg : Gain  Gain=180/pi  SaturateOnIntegerOverflow=on  OutDataTypeStr=Inherit: Same as input  ParamDataTypeStr=Inherit: Same as input
  Conversion Rotation to Angle : Gain  Gain=2*pi  SaturateOnIntegerOverflow=on  OutDataTypeStr=Inherit: Same as input  ParamDataTypeStr=Inherit: Same as input
  Dead Zone : DeadZone  LowerValue=-5000  UpperValue=5000  SaturateOnIntegerOverflow=on
  Derivative : Derivative
  Gear : Gain  Gain=6.33e-3  SaturateOnIntegerOverflow=on  OutDataTypeStr=Inherit: Same as input  ParamDataTypeStr=Inherit: Same as input
  Init Angle : Switch  Threshold=1  SaturateOnIntegerOverflow=on  InputSameDT=on
  Memory : Memory
  Memory1 : Memory
  Mux : Mux  Inputs=2
  Product : Product  SaturateOnIntegerOverflow=on  RndMeth=Zero  InputSameDT=on  OutDataTypeStr=Inherit: Same as first input
  Saturation : Saturate  UpperLimit=1  LowerLimit=-1
  Sum : Sum  Inputs=+-  SaturateOnIntegerOverflow=on  InputSameDT=on  OutDataTypeStr=Inherit: Same as first input
  Sum1 : Sum  Inputs=++-  SaturateOnIntegerOverflow=on  InputSameDT=on  OutDataTypeStr=Inherit: Same as first input
  Position : Outport
  wires:
  Gear/1 -> Conversion Rad to Deg/1
  Sum1/1 -> Gear/1
  Sum/1 -> Product/1
  Dead Zone/1 -> Saturation/1
  Derivative/1 -> Dead Zone/1
  Mux/1 -> Atan2/1
  Sin/1 -> Mux/1
  Conversion Rad to Deg/1 -> Position/1
  Saturation/1 -> Sum/2
  Conversion Rotation to Angle/1 -> Sum1/1
  Reset (Impulse)/1 -> Product/2, Init Angle/2
  Atan2/1 -> Derivative/1, Sum1/2, Init Angle/3
  Cos/1 -> Mux/2
  Memory/1 -> Sum/1
  Product/1 -> Conversion Rotation to Angle/1, Memory/1
  Memory1/1 -> Init Angle/1
  Init Angle/1 -> Sum1/3, Memory1/1

== system main/Position 2/Filters 2 ==
  Sin && Cos : Inport
  Analog Butterworth LP Filter : Subsystem  mask(buttap){Parameter3=2*pi*16, Parameter4=1}
      mask prompts: Parameter3 "Cutoff frequency (rad/sec)"; Parameter4 "Order"
      mask help:
      | Analog Butterworth low pass filter.
      |
      | (Requires Signal Processing Toolbox)
      mask init:
      | [z,p,k]=buttap(@2); z=@1*z; p=@1*p; k=real(prod(-p)); [num,den]=zp2tf(z,p,k); w=logspace(log10(@1/10),log10(10*@1),20); h=freqs(num,den,w);
      mask Help: Butterworth low pass filter using MATLAB's butter command.
      mask Display: plot(20*log10(w),20*log10(abs(h)))
  Analog Butterworth LP Filter1 : Subsystem  mask(buttap){Parameter3=2*pi*16, Parameter4=1}
      mask prompts: Parameter3 "Cutoff frequency (rad/sec)"; Parameter4 "Order"
      mask help:
      | Analog Butterworth low pass filter.
      |
      | (Requires Signal Processing Toolbox)
      mask init:
      | [z,p,k]=buttap(@2); z=@1*z; p=@1*p; k=real(prod(-p)); [num,den]=zp2tf(z,p,k); w=logspace(log10(@1/10),log10(10*@1),20); h=freqs(num,den,w);
      mask Help: Butterworth low pass filter using MATLAB's butter command.
      mask Display: plot(20*log10(w),20*log10(abs(h)))
  Demux : Demux  Outputs=2
  Sin : Outport
  Cos : Outport  Port=2
  wires:
  Analog Butterworth LP Filter/1(Out1) -> Sin/1
  Analog Butterworth LP Filter1/1(Out1) -> Cos/1
  Sin && Cos/1 -> Demux/1
  Demux/1 -> Analog Butterworth LP Filter/1(In1)
  Demux/2 -> Analog Butterworth LP Filter1/1(In1)

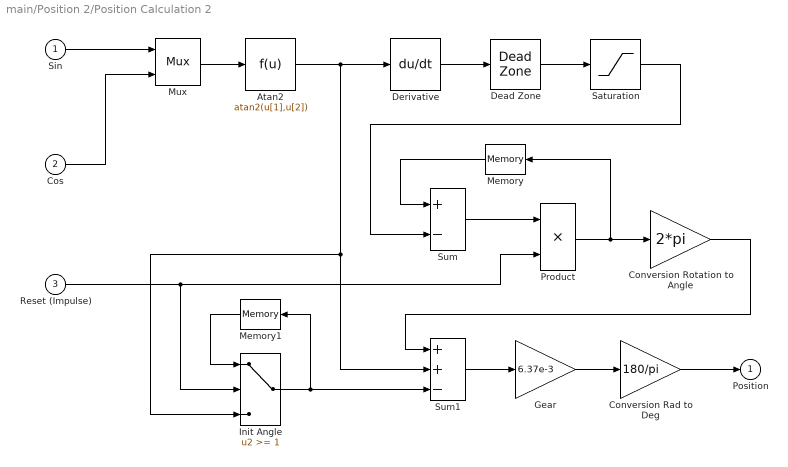
== system main/Position 2/Position Calculation 2 ==
  Sin : Inport
  Cos : Inport  Port=2
  Reset (Impulse) : Inport  Port=3
  Atan2 : Fcn  Expr=atan2(u[1],u[2])
  Conversion Rad to Deg : Gain  Gain=180/pi  SaturateOnIntegerOverflow=on  OutDataTypeStr=Inherit: Same as input  ParamDataTypeStr=Inherit: Same as input
  Conversion Rotation to Angle : Gain  Gain=2*pi  SaturateOnIntegerOverflow=on  OutDataTypeStr=Inherit: Same as input  ParamDataTypeStr=Inherit: Same as input
  Dead Zone : DeadZone  LowerValue=-5000  UpperValue=5000  SaturateOnIntegerOverflow=on
  Derivative : Derivative
  Gear : Gain  Gain=6.37e-3  SaturateOnIntegerOverflow=on  OutDataTypeStr=Inherit: Same as input  ParamDataTypeStr=Inherit: Same as input
  Init Angle : Switch  Threshold=1  SaturateOnIntegerOverflow=on  InputSameDT=on
  Memory : Memory
  Memory1 : Memory
  Mux : Mux  Inputs=2
  Product : Product  SaturateOnIntegerOverflow=on  RndMeth=Zero  InputSameDT=on  OutDataTypeStr=Inherit: Same as first input
  Saturation : Saturate  UpperLimit=1  LowerLimit=-1
  Sum : Sum  Inputs=+-  SaturateOnIntegerOverflow=on  InputSameDT=on  OutDataTypeStr=Inherit: Same as first input
  Sum1 : Sum  Inputs=++-  SaturateOnIntegerOverflow=on  InputSameDT=on  OutDataTypeStr=Inherit: Same as first input
  Position : Outport
  wires:
  Gear/1 -> Conversion Rad to Deg/1
  Sum1/1 -> Gear/1
  Sum/1 -> Product/1
  Dead Zone/1 -> Saturation/1
  Derivative/1 -> Dead Zone/1
  Mux/1 -> Atan2/1
  Sin/1 -> Mux/1
  Conversion Rad to Deg/1 -> Position/1
  Saturation/1 -> Sum/2
  Conversion Rotation to Angle/1 -> Sum1/1
  Reset (Impulse)/1 -> Product/2, Init Angle/2
  Atan2/1 -> Derivative/1, Sum1/2, Init Angle/3
  Cos/1 -> Mux/2
  Memory/1 -> Sum/1
  Product/1 -> Conversion Rotation to Angle/1, Memory/1
  Memory1/1 -> Init Angle/1
  Init Angle/1 -> Sum1/3, Memory1/1

== system main/Position 3/Filters 3 ==
  Sin && Cos : Inport
  Analog Butterworth LP Filter : Subsystem  mask(buttap){Parameter3=2*pi*16, Parameter4=1}
      mask prompts: Parameter3 "Cutoff frequency (rad/sec)"; Parameter4 "Order"
      mask help:
      | Analog Butterworth low pass filter.
      |
      | (Requires Signal Processing Toolbox)
      mask init:
      | [z,p,k]=buttap(@2); z=@1*z; p=@1*p; k=real(prod(-p)); [num,den]=zp2tf(z,p,k); w=logspace(log10(@1/10),log10(10*@1),20); h=freqs(num,den,w);
      mask Help: Butterworth low pass filter using MATLAB's butter command.
      mask Display: plot(20*log10(w),20*log10(abs(h)))
  Analog Butterworth LP Filter1 : Subsystem  mask(buttap){Parameter3=2*pi*16, Parameter4=1}
      mask prompts: Parameter3 "Cutoff frequency (rad/sec)"; Parameter4 "Order"
      mask help:
      | Analog Butterworth low pass filter.
      |
      | (Requires Signal Processing Toolbox)
      mask init:
      | [z,p,k]=buttap(@2); z=@1*z; p=@1*p; k=real(prod(-p)); [num,den]=zp2tf(z,p,k); w=logspace(log10(@1/10),log10(10*@1),20); h=freqs(num,den,w);
      mask Help: Butterworth low pass filter using MATLAB's butter command.
      mask Display: plot(20*log10(w),20*log10(abs(h)))
  Demux : Demux  Outputs=2
  Sin : Outport
  Cos : Outport  Port=2
  wires:
  Analog Butterworth LP Filter/1(Out1) -> Sin/1
  Analog Butterworth LP Filter1/1(Out1) -> Cos/1
  Sin && Cos/1 -> Demux/1
  Demux/1 -> Analog Butterworth LP Filter/1(In1)
  Demux/2 -> Analog Butterworth LP Filter1/1(In1)

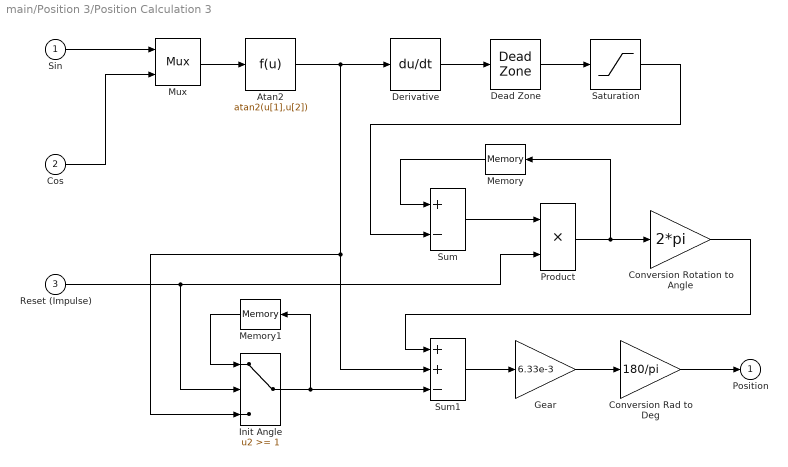
== system main/Position 3/Position Calculation 3 ==
  Sin : Inport
  Cos : Inport  Port=2
  Reset (Impulse) : Inport  Port=3
  Atan2 : Fcn  Expr=atan2(u[1],u[2])
  Conversion Rad to Deg : Gain  Gain=180/pi  SaturateOnIntegerOverflow=on  OutDataTypeStr=Inherit: Same as input  ParamDataTypeStr=Inherit: Same as input
  Conversion Rotation to Angle : Gain  Gain=2*pi  SaturateOnIntegerOverflow=on  OutDataTypeStr=Inherit: Same as input  ParamDataTypeStr=Inherit: Same as input
  Dead Zone : DeadZone  LowerValue=-5000  UpperValue=5000  SaturateOnIntegerOverflow=on
  Derivative : Derivative
  Gear : Gain  Gain=6.33e-3  SaturateOnIntegerOverflow=on  OutDataTypeStr=Inherit: Same as input  ParamDataTypeStr=Inherit: Same as input
  Init Angle : Switch  Threshold=1  SaturateOnIntegerOverflow=on  InputSameDT=on
  Memory : Memory
  Memory1 : Memory
  Mux : Mux  Inputs=2
  Product : Product  SaturateOnIntegerOverflow=on  RndMeth=Zero  InputSameDT=on  OutDataTypeStr=Inherit: Same as first input
  Saturation : Saturate  UpperLimit=1  LowerLimit=-1
  Sum : Sum  Inputs=+-  SaturateOnIntegerOverflow=on  InputSameDT=on  OutDataTypeStr=Inherit: Same as first input
  Sum1 : Sum  Inputs=++-  SaturateOnIntegerOverflow=on  InputSameDT=on  OutDataTypeStr=Inherit: Same as first input
  Position : Outport
  wires:
  Gear/1 -> Conversion Rad to Deg/1
  Sum1/1 -> Gear/1
  Sum/1 -> Product/1
  Dead Zone/1 -> Saturation/1
  Derivative/1 -> Dead Zone/1
  Mux/1 -> Atan2/1
  Sin/1 -> Mux/1
  Conversion Rad to Deg/1 -> Position/1
  Saturation/1 -> Sum/2
  Conversion Rotation to Angle/1 -> Sum1/1
  Reset (Impulse)/1 -> Product/2, Init Angle/2
  Atan2/1 -> Derivative/1, Sum1/2, Init Angle/3
  Cos/1 -> Mux/2
  Memory/1 -> Sum/1
  Product/1 -> Conversion Rotation to Angle/1, Memory/1
  Memory1/1 -> Init Angle/1
  Init Angle/1 -> Sum1/3, Memory1/1

== system main/Position 4/Filters 4 ==
  Sin && Cos : Inport
  Analog Butterworth LP Filter : Subsystem  mask(buttap){Parameter3=2*pi*16, Parameter4=1}
      mask prompts: Parameter3 "Cutoff frequency (rad/sec)"; Parameter4 "Order"
      mask help:
      | Analog Butterworth low pass filter.
      |
      | (Requires Signal Processing Toolbox)
      mask init:
      | [z,p,k]=buttap(@2); z=@1*z; p=@1*p; k=real(prod(-p)); [num,den]=zp2tf(z,p,k); w=logspace(log10(@1/10),log10(10*@1),20); h=freqs(num,den,w);
      mask Help: Butterworth low pass filter using MATLAB's butter command.
      mask Display: plot(20*log10(w),20*log10(abs(h)))
  Analog Butterworth LP Filter1 : Subsystem  mask(buttap){Parameter3=2*pi*16, Parameter4=1}
      mask prompts: Parameter3 "Cutoff frequency (rad/sec)"; Parameter4 "Order"
      mask help:
      | Analog Butterworth low pass filter.
      |
      | (Requires Signal Processing Toolbox)
      mask init:
      | [z,p,k]=buttap(@2); z=@1*z; p=@1*p; k=real(prod(-p)); [num,den]=zp2tf(z,p,k); w=logspace(log10(@1/10),log10(10*@1),20); h=freqs(num,den,w);
      mask Help: Butterworth low pass filter using MATLAB's butter command.
      mask Display: plot(20*log10(w),20*log10(abs(h)))
  Demux : Demux  Outputs=2
  Sin : Outport
  Cos : Outport  Port=2
  wires:
  Demux/2 -> Analog Butterworth LP Filter1/1(In1)
  Demux/1 -> Analog Butterworth LP Filter/1(In1)
  Sin && Cos/1 -> Demux/1
  Analog Butterworth LP Filter1/1(Out1) -> Cos/1
  Analog Butterworth LP Filter/1(Out1) -> Sin/1

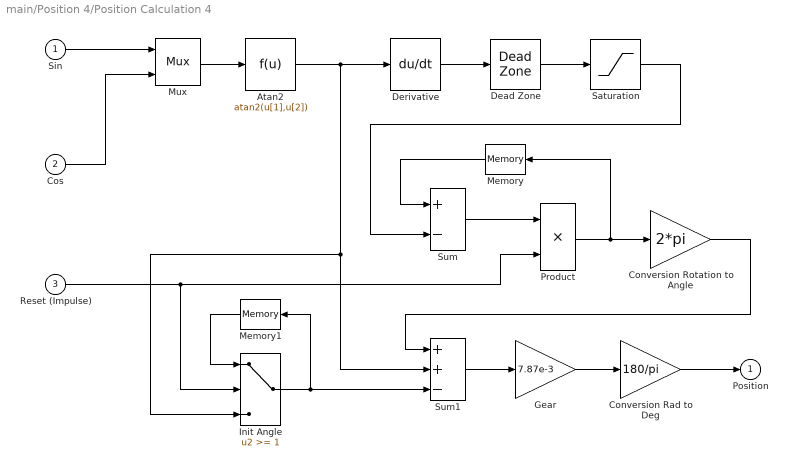
== system main/Position 4/Position Calculation 4 ==
  Sin : Inport
  Cos : Inport  Port=2
  Reset (Impulse) : Inport  Port=3
  Atan2 : Fcn  Expr=atan2(u[1],u[2])
  Conversion Rad to Deg : Gain  Gain=180/pi  SaturateOnIntegerOverflow=on  OutDataTypeStr=Inherit: Same as input  ParamDataTypeStr=Inherit: Same as input
  Conversion Rotation to Angle : Gain  Gain=2*pi  SaturateOnIntegerOverflow=on  OutDataTypeStr=Inherit: Same as input  ParamDataTypeStr=Inherit: Same as input
  Dead Zone : DeadZone  LowerValue=-5000  UpperValue=5000  SaturateOnIntegerOverflow=on
  Derivative : Derivative
  Gear : Gain  Gain=7.87e-3  SaturateOnIntegerOverflow=on  OutDataTypeStr=Inherit: Same as input  ParamDataTypeStr=Inherit: Same as input
  Init Angle : Switch  Threshold=1  SaturateOnIntegerOverflow=on  InputSameDT=on
  Memory : Memory
  Memory1 : Memory
  Mux : Mux  Inputs=2
  Product : Product  SaturateOnIntegerOverflow=on  RndMeth=Zero  InputSameDT=on  OutDataTypeStr=Inherit: Same as first input
  Saturation : Saturate  UpperLimit=1  LowerLimit=-1
  Sum : Sum  Inputs=+-  SaturateOnIntegerOverflow=on  InputSameDT=on  OutDataTypeStr=Inherit: Same as first input
  Sum1 : Sum  Inputs=++-  SaturateOnIntegerOverflow=on  InputSameDT=on  OutDataTypeStr=Inherit: Same as first input
  Position : Outport
  wires:
  Init Angle/1 -> Memory1/1, Sum1/3
  Memory1/1 -> Init Angle/1
  Product/1 -> Memory/1, Conversion Rotation to Angle/1
  Memory/1 -> Sum/1
  Cos/1 -> Mux/2
  Atan2/1 -> Init Angle/3, Sum1/2, Derivative/1
  Reset (Impulse)/1 -> Init Angle/2, Product/2
  Conversion Rotation to Angle/1 -> Sum1/1
  Saturation/1 -> Sum/2
  Conversion Rad to Deg/1 -> Position/1
  Sin/1 -> Mux/1
  Mux/1 -> Atan2/1
  Derivative/1 -> Dead Zone/1
  Dead Zone/1 -> Saturation/1
  Sum/1 -> Product/1
  Sum1/1 -> Gear/1
  Gear/1 -> Conversion Rad to Deg/1

== system main/Position 5/Filters 5 ==
  Sin && Cos : Inport
  Analog Butterworth LP Filter : Subsystem  mask(buttap){Parameter3=2*pi*16, Parameter4=1}
      mask prompts: Parameter3 "Cutoff frequency (rad/sec)"; Parameter4 "Order"
      mask help:
      | Analog Butterworth low pass filter.
      |
      | (Requires Signal Processing Toolbox)
      mask init:
      | [z,p,k]=buttap(@2); z=@1*z; p=@1*p; k=real(prod(-p)); [num,den]=zp2tf(z,p,k); w=logspace(log10(@1/10),log10(10*@1),20); h=freqs(num,den,w);
      mask Help: Butterworth low pass filter using MATLAB's butter command.
      mask Display: plot(20*log10(w),20*log10(abs(h)))
  Analog Butterworth LP Filter1 : Subsystem  mask(buttap){Parameter3=2*pi*16, Parameter4=1}
      mask prompts: Parameter3 "Cutoff frequency (rad/sec)"; Parameter4 "Order"
      mask help:
      | Analog Butterworth low pass filter.
      |
      | (Requires Signal Processing Toolbox)
      mask init:
      | [z,p,k]=buttap(@2); z=@1*z; p=@1*p; k=real(prod(-p)); [num,den]=zp2tf(z,p,k); w=logspace(log10(@1/10),log10(10*@1),20); h=freqs(num,den,w);
      mask Help: Butterworth low pass filter using MATLAB's butter command.
      mask Display: plot(20*log10(w),20*log10(abs(h)))
  Demux : Demux  Outputs=2
  Sin : Outport
  Cos : Outport  Port=2
  wires:
  Demux/2 -> Analog Butterworth LP Filter1/1(In1)
  Demux/1 -> Analog Butterworth LP Filter/1(In1)
  Sin && Cos/1 -> Demux/1
  Analog Butterworth LP Filter1/1(Out1) -> Cos/1
  Analog Butterworth LP Filter/1(Out1) -> Sin/1

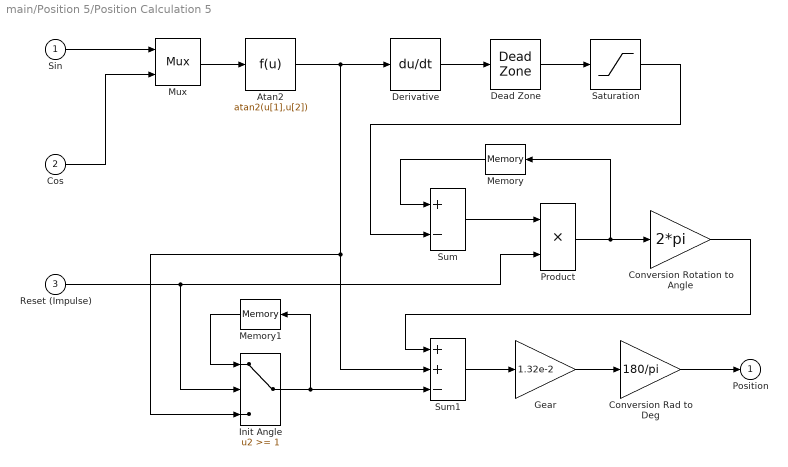
== system main/Position 5/Position Calculation 5 ==
  Sin : Inport
  Cos : Inport  Port=2
  Reset (Impulse) : Inport  Port=3
  Atan2 : Fcn  Expr=atan2(u[1],u[2])
  Conversion Rad to Deg : Gain  Gain=180/pi  SaturateOnIntegerOverflow=on  OutDataTypeStr=Inherit: Same as input  ParamDataTypeStr=Inherit: Same as input
  Conversion Rotation to Angle : Gain  Gain=2*pi  SaturateOnIntegerOverflow=on  OutDataTypeStr=Inherit: Same as input  ParamDataTypeStr=Inherit: Same as input
  Dead Zone : DeadZone  LowerValue=-5000  UpperValue=5000  SaturateOnIntegerOverflow=on
  Derivative : Derivative
  Gear : Gain  Gain=1.32e-2  SaturateOnIntegerOverflow=on  OutDataTypeStr=Inherit: Same as input  ParamDataTypeStr=Inherit: Same as input
  Init Angle : Switch  Threshold=1  SaturateOnIntegerOverflow=on  InputSameDT=on
  Memory : Memory
  Memory1 : Memory
  Mux : Mux  Inputs=2
  Product : Product  SaturateOnIntegerOverflow=on  RndMeth=Zero  InputSameDT=on  OutDataTypeStr=Inherit: Same as first input
  Saturation : Saturate  UpperLimit=1  LowerLimit=-1
  Sum : Sum  Inputs=+-  SaturateOnIntegerOverflow=on  InputSameDT=on  OutDataTypeStr=Inherit: Same as first input
  Sum1 : Sum  Inputs=++-  SaturateOnIntegerOverflow=on  InputSameDT=on  OutDataTypeStr=Inherit: Same as first input
  Position : Outport
  wires:
  Init Angle/1 -> Memory1/1, Sum1/3
  Memory1/1 -> Init Angle/1
  Product/1 -> Memory/1, Conversion Rotation to Angle/1
  Memory/1 -> Sum/1
  Cos/1 -> Mux/2
  Atan2/1 -> Init Angle/3, Sum1/2, Derivative/1
  Reset (Impulse)/1 -> Init Angle/2, Product/2
  Conversion Rotation to Angle/1 -> Sum1/1
  Saturation/1 -> Sum/2
  Conversion Rad to Deg/1 -> Position/1
  Sin/1 -> Mux/1
  Mux/1 -> Atan2/1
  Derivative/1 -> Dead Zone/1
  Dead Zone/1 -> Saturation/1
  Sum/1 -> Product/1
  Sum1/1 -> Gear/1
  Gear/1 -> Conversion Rad to Deg/1

== system main/RTI Data/RTI Data Store ==
  RTI Data Store : Subsystem  mask(RTI_DATA_STORE){}
      mask help:
      | RTI Data Store Block. This block is used by RTI to store internal model dependent data. Deleting this block will result in data loss.
      |
      | NEVER DELETE, COPY, OR MODIFY THIS BLOCK!
      mask Help:
      | RTI Data Store Block. This block is used by RTI to store internal model dependent data. Deleting this block will result in data loss.
      | 
      | NEVER DELETE, COPY, OR MODIFY THIS BLOCK!
      mask Display: text(0.5, 0.5, ' ', 'HorizontalAlignment', 'center');

== system main/Position 1/Filters 1/Analog Butterworth LP Filter ==
  In1 : Inport
  Analog Butterworth LP Filter : ZeroPole  Zeros=z  Poles=p  Gain=k
  Out1 : Outport
  wires:
  In1/1 -> Analog Butterworth LP Filter/1
  Analog Butterworth LP Filter/1 -> Out1/1

== system main/Position 1/Filters 1/Analog Butterworth LP Filter1 ==
  In1 : Inport
  Analog Butterworth LP Filter1 : ZeroPole  Zeros=z  Poles=p  Gain=k
  Out1 : Outport
  wires:
  In1/1 -> Analog Butterworth LP Filter1/1
  Analog Butterworth LP Filter1/1 -> Out1/1

== system main/Position 2/Filters 2/Analog Butterworth LP Filter ==
  In1 : Inport
  Analog Butterworth LP Filter : ZeroPole  Zeros=z  Poles=p  Gain=k
  Out1 : Outport
  wires:
  In1/1 -> Analog Butterworth LP Filter/1
  Analog Butterworth LP Filter/1 -> Out1/1

== system main/Position 2/Filters 2/Analog Butterworth LP Filter1 ==
  In1 : Inport
  Analog Butterworth LP Filter1 : ZeroPole  Zeros=z  Poles=p  Gain=k
  Out1 : Outport
  wires:
  In1/1 -> Analog Butterworth LP Filter1/1
  Analog Butterworth LP Filter1/1 -> Out1/1

== system main/Position 3/Filters 3/Analog Butterworth LP Filter ==
  In1 : Inport
  Analog Butterworth LP Filter : ZeroPole  Zeros=z  Poles=p  Gain=k
  Out1 : Outport
  wires:
  In1/1 -> Analog Butterworth LP Filter/1
  Analog Butterworth LP Filter/1 -> Out1/1

== system main/Position 3/Filters 3/Analog Butterworth LP Filter1 ==
  In1 : Inport
  Analog Butterworth LP Filter1 : ZeroPole  Zeros=z  Poles=p  Gain=k
  Out1 : Outport
  wires:
  In1/1 -> Analog Butterworth LP Filter1/1
  Analog Butterworth LP Filter1/1 -> Out1/1

== system main/Position 4/Filters 4/Analog Butterworth LP Filter ==
  In1 : Inport
  Analog Butterworth LP Filter : ZeroPole  Zeros=z  Poles=p  Gain=k
  Out1 : Outport
  wires:
  In1/1 -> Analog Butterworth LP Filter/1
  Analog Butterworth LP Filter/1 -> Out1/1

== system main/Position 4/Filters 4/Analog Butterworth LP Filter1 ==
  In1 : Inport
  Analog Butterworth LP Filter1 : ZeroPole  Zeros=z  Poles=p  Gain=k
  Out1 : Outport
  wires:
  In1/1 -> Analog Butterworth LP Filter1/1
  Analog Butterworth LP Filter1/1 -> Out1/1

== system main/Position 5/Filters 5/Analog Butterworth LP Filter ==
  In1 : Inport
  Analog Butterworth LP Filter : ZeroPole  Zeros=z  Poles=p  Gain=k
  Out1 : Outport
  wires:
  In1/1 -> Analog Butterworth LP Filter/1
  Analog Butterworth LP Filter/1 -> Out1/1

== system main/Position 5/Filters 5/Analog Butterworth LP Filter1 ==
  In1 : Inport
  Analog Butterworth LP Filter1 : ZeroPole  Zeros=z  Poles=p  Gain=k
  Out1 : Outport
  wires:
  In1/1 -> Analog Butterworth LP Filter1/1
  Analog Butterworth LP Filter1/1 -> Out1/1

== system main/RTI Data/RTI Data Store/RTI Data Store ==
  RTI Data Store : Subsystem  mask(RTI_DATA_STORE){}
      mask help:
      | RTI Data Store Block. This block is used by RTI to store internal model dependent data. Deleting this block will result in data loss.
      |
      | NEVER DELETE, COPY, OR MODIFY THIS BLOCK!
      mask Help:
      | RTI Data Store Block. This block is used by RTI to store internal model dependent data. Deleting this block will result in data loss.
      | 
      | NEVER DELETE, COPY, OR MODIFY THIS BLOCK!
      mask Display: text(0.5, 0.5, ' ', 'HorizontalAlignment', 'center');

== system main/RTI Data/RTI Data Store/RTI Data Store/RTI Data Store ==
  RTI Data Store : Subsystem  mask(RTI_DATA_STORE){}
      mask help:
      | RTI Data Store Block. This block is used by RTI to store internal model dependent data. Deleting this block will result in data loss.
      |
      | NEVER DELETE, COPY, OR MODIFY THIS BLOCK!
      mask Help:
      | RTI Data Store Block. This block is used by RTI to store internal model dependent data. Deleting this block will result in data loss.
      | 
      | NEVER DELETE, COPY, OR MODIFY THIS BLOCK!
      mask Display: text(0.5, 0.5, ' ', 'HorizontalAlignment', 'center');

== system main/RTI Data/RTI Data Store/RTI Data Store/RTI Data Store/RTI Data Store ==
